simulink model "TP1_P2_3_Q6_D"  (R2024b)
settings: Solver=VariableStepAuto  StartTime=0.0  StopTime=10.0  RelTol=1e-9  AbsTol=1e-9
values from neighbouring files (symbols this model uses):
  K = (4*Jeff)/((e.^2)*(KR))    [sf_loi_avant_RP.m]    (also in sf_retour_linearisant_boucle_interne_RP.m; valeurs.m)
  Kd = ((4*Jeff)/(1/2) - Beff)/KR    (= 0.235)    [sf_loi_avant_RP.m]    (also in sf_retour_linearisant_boucle_interne_RP.m = 400.225; valeurs.m = 400.225)
  r = 1/200    (= 0.005)    [sf_loi_avant_RP.m]    (also in sf_retour_linearisant_boucle_interne_RP.m = 1; valeurs.m = 1)
  Ti = 0.8    [sf_loi_avant_RP.m]    (also in sf_retour_linearisant_boucle_interne_RP.m; valeurs.m = 1)
libraries: lib_robotRP x2
settings Model: Creator=GWC4238A
settings RTWCC: GPUComputeCapability=3.5

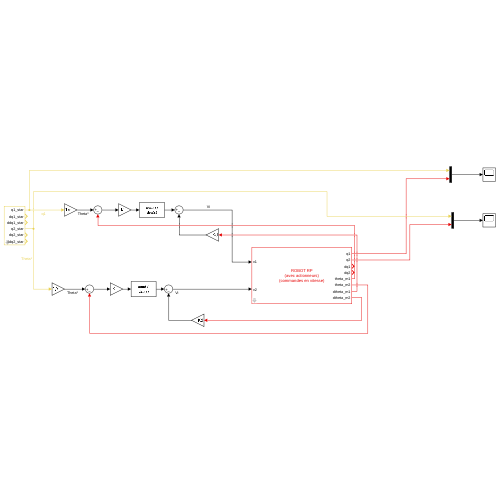
[thumbnail: Simulink's stored preview of the top-level diagram]
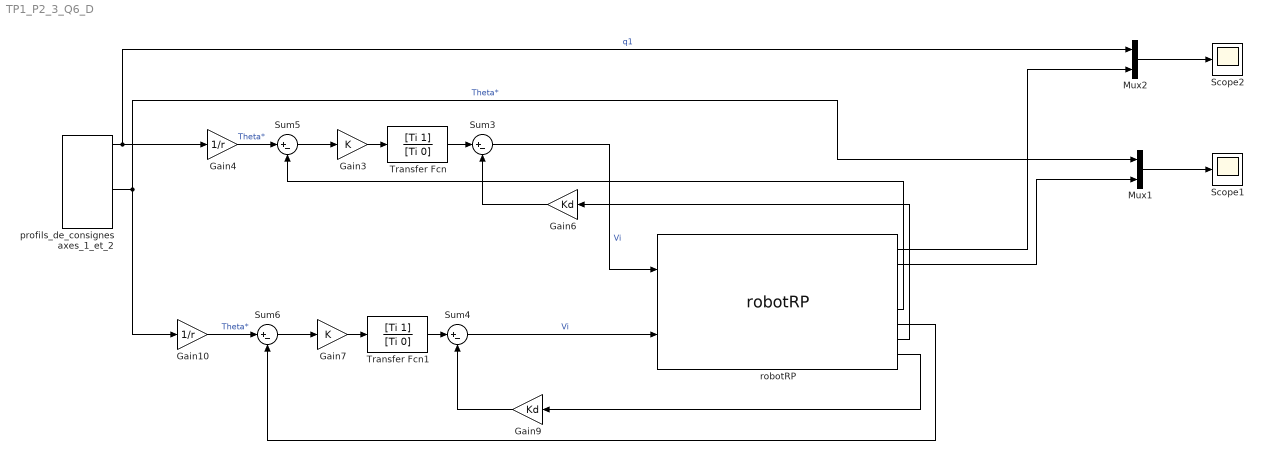
== system TP1_P2_3_Q6_D ==
  Gain10 : Gain  Gain=1/r
  Gain3 : Gain  Gain=K
  Gain4 : Gain  Gain=1/r
  Gain6 : Gain  Gain=Kd
  Gain7 : Gain  Gain=K
  Gain9 : Gain  Gain=Kd
  Mux1 : Mux  Inputs=2
  Mux2 : Mux  Inputs=2
  Scope1 : Scope
  Scope2 : Scope
  Sum{3..6} (4 alike) : Sum  Inputs=|+-
  Transfer Fcn : TransferFcn  Numerator=[Ti 1]  Denominator=[Ti 0]
  Transfer Fcn1 : TransferFcn  Numerator=[Ti 1]  Denominator=[Ti 0]
  profils_de_consignes axes_1_et_2 : lib_robotRP/profils_de_consignes axes_1_et_2
  robotRP : lib_robotRP/robotRP  vecteur_theta_dtheta_initial=[0 ; 0.5/r ; 0 ; 0]  m=15  gX=0  gY=-9.81  F1=0  F2=0  H1=0  H2=0  Km_sur_R=0.3  Jm=0.01  Beff=0.0125  r=r
  wires:
  profils_de_consignes axes_1_et_2/1 -> Gain4/1, Mux2/1  "q1"
  robotRP/8 -> Gain9/1
  robotRP/6 -> Sum6/2
  Mux1/1 -> Scope1/1
  Mux2/1 -> Scope2/1
  robotRP/1 -> Mux2/2
  robotRP/2 -> Mux1/2
  Transfer Fcn/1 -> Sum3/1
  Sum3/1 -> robotRP/1  "Vi"
  Gain6/1 -> Sum3/2
  Sum5/1 -> Gain3/1
  robotRP/7 -> Gain6/1
  robotRP/5 -> Sum5/2
  Gain4/1 -> Sum5/1  "Theta*"
  Sum6/1 -> Gain7/1
  Gain7/1 -> Transfer Fcn1/1
  Sum4/1 -> robotRP/2  "Vi"
  profils_de_consignes axes_1_et_2/4 -> Gain10/1, Mux1/1  "Theta*"
  Gain9/1 -> Sum4/2
  Gain10/1 -> Sum6/1  "Theta*"
  Gain3/1 -> Transfer Fcn/1
  Transfer Fcn1/1 -> Sum4/1
